simulink model "PID"  (R2019a)
settings: configuration reference "Configuration" (kept outside this file)
undefined symbols (not defined in the file): DiscIntNeverNeededParam, Model_Param
settings Model: Creator=zouji  LastModifiedBy=Bingo
settings ConfigSetRef: SourceName=Configuration  SourceLocation=Base Workspace

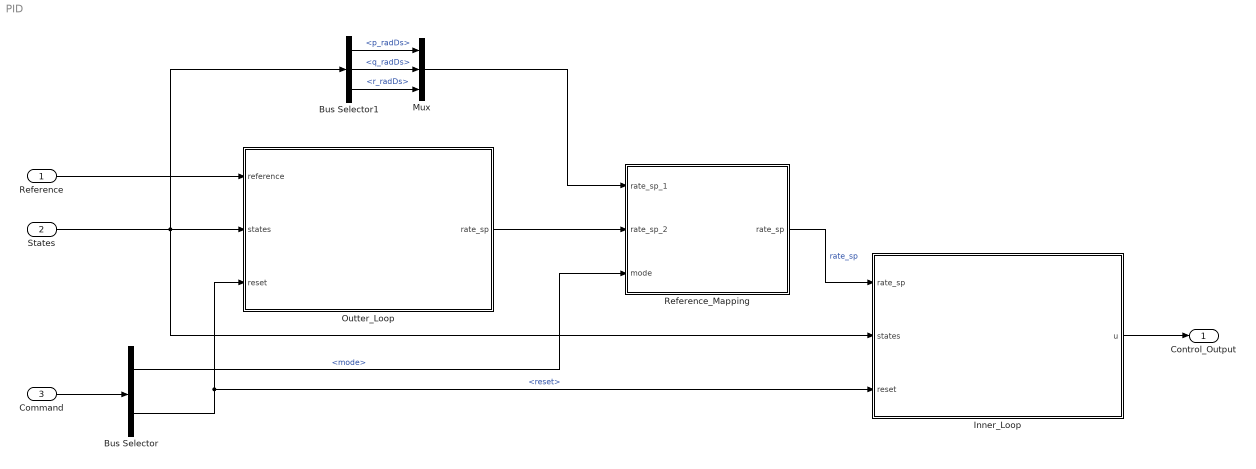
== system PID ==
  Reference : Inport  OutDataTypeStr=Bus: Reference
  States : Inport  Port=2  OutDataTypeStr=Bus: States
  Command : Inport  Port=3  OutDataTypeStr=Bus: Command
  Bus Selector : BusSelector  OutputSignals=mode,reset
  Bus Selector1 : BusSelector  OutputSignals=p_radDs,q_radDs,r_radDs
  Inner_Loop : Subsystem
  Mux : Mux  Inputs=3
  Outter_Loop : Subsystem
  Reference_Mapping : Subsystem
  Control_Output : Outport  OutDataTypeStr=Bus: Control_Output
  wires:
  Command/1 -> Bus Selector/1
  Reference/1 -> Outter_Loop/1(reference)
  States/1 -> Bus Selector1/1, Outter_Loop/2(states), Inner_Loop/2(states)
  Inner_Loop/1(u) -> Control_Output/1
  Bus Selector/2 -> Inner_Loop/3(reset), Outter_Loop/3(reset)  "<reset>"
  Reference_Mapping/1(rate_sp) -> Inner_Loop/1(rate_sp)  "rate_sp"
  Outter_Loop/1(rate_sp) -> Reference_Mapping/2(rate_sp_2)
  Bus Selector1/1 -> Mux/1  "<p_radDs>"
  Bus Selector1/2 -> Mux/2  "<q_radDs>"
  Bus Selector1/3 -> Mux/3  "<r_radDs>"
  Mux/1 -> Reference_Mapping/1(rate_sp_1)
  Bus Selector/1 -> Reference_Mapping/3(mode)  "<mode>"

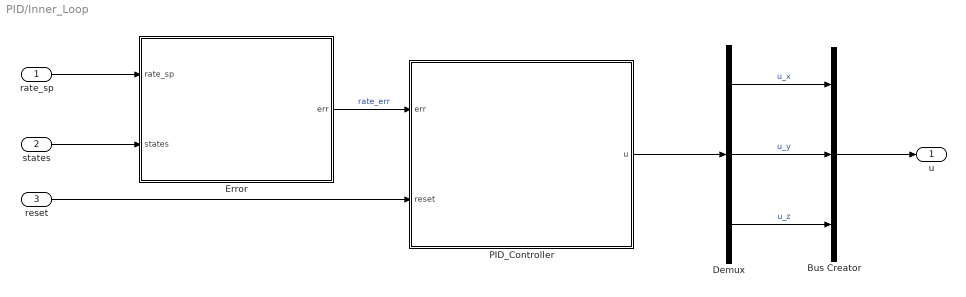
== system PID/Inner_Loop ==
  rate_sp : Inport
  states : Inport  Port=2
  reset : Inport  Port=3
  Bus Creator : BusCreator  Inputs=3
  Demux : Demux  Outputs=3
  Error : Subsystem
  PID_Controller : Subsystem
  u : Outport  OutDataTypeStr=Bus: Control_Output
  wires:
  states/1 -> Error/2(states)
  Error/1(err) -> PID_Controller/1(err)  "rate_err"
  rate_sp/1 -> Error/1(rate_sp)
  reset/1 -> PID_Controller/2(reset)
  PID_Controller/1(u) -> Demux/1
  Demux/1 -> Bus Creator/1  "u_x"
  Demux/2 -> Bus Creator/2  "u_y"
  Demux/3 -> Bus Creator/3  "u_z"
  Bus Creator/1 -> u/1

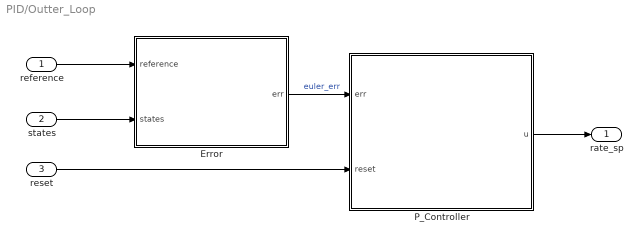
== system PID/Outter_Loop ==
  reference : Inport
  states : Inport  Port=2
  reset : Inport  Port=3
  Error : Subsystem
  P_Controller : Subsystem
  rate_sp : Outport
  wires:
  states/1 -> Error/2(states)
  Error/1(err) -> P_Controller/1(err)  "euler_err"
  P_Controller/1(u) -> rate_sp/1
  reset/1 -> P_Controller/2(reset)
  reference/1 -> Error/1(reference)

== system PID/Reference_Mapping ==
  note: mode=0, 外环输出作为目标角速度
      | mode=1, 输入指令作为目标角速度
  rate_sp_1 : Inport
  rate_sp_2 : Inport  Port=2
  mode : Inport  Port=3
  Switch : Switch  Criteria=u2 > Threshold
  rate_sp : Outport
  wires:
  mode/1 -> Switch/2
  rate_sp_1/1 -> Switch/1
  rate_sp_2/1 -> Switch/3
  Switch/1 -> rate_sp/1

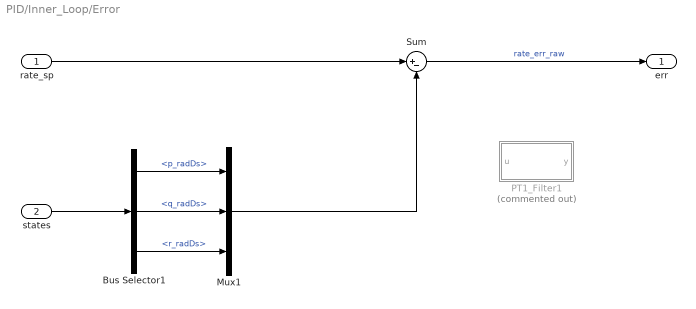
== system PID/Inner_Loop/Error ==
  rate_sp : Inport
  states : Inport  Port=2
  Bus Selector1 : BusSelector  OutputSignals=p_radDs,q_radDs,r_radDs
  Mux1 : Mux  Inputs=3
  PT1_Filter1 : Subsystem  Commented=on  mask{T_filter=0.05}
      mask prompts: T_filter "Time constant [s]"
      mask Display: fprintf('T = %.3f', T_filter)
  Sum : Sum  Inputs=|+-
  err : Outport
  wires:
  Bus Selector1/2 -> Mux1/2  "<q_radDs>"
  Bus Selector1/3 -> Mux1/3  "<r_radDs>"
  Bus Selector1/1 -> Mux1/1  "<p_radDs>"
  states/1 -> Bus Selector1/1
  Mux1/1 -> Sum/2
  Sum/1 -> err/1  "rate_err_raw"
  rate_sp/1 -> Sum/1

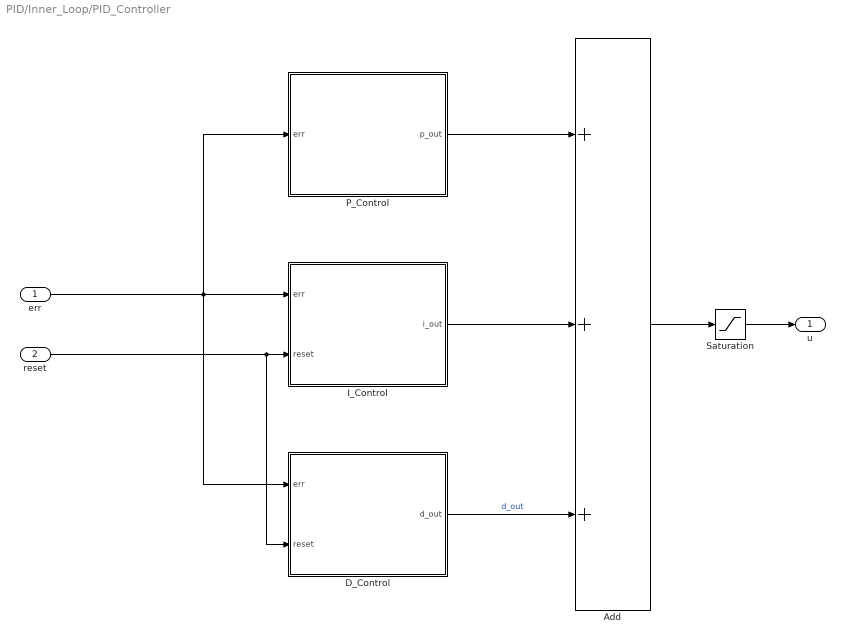
== system PID/Inner_Loop/PID_Controller ==
  err : Inport
  reset : Inport  Port=2
  Add : Sum  Inputs=+++
  D_Control : Subsystem  mask{p_kd=Model_Param.Kd_p, q_kd=Model_Param.Kd_q, r_kd=Model_Param.Kd_r, max_d=Model_Param.Kd_Max, min_d=Model_Param.Kd_Min}
  I_Control : Subsystem  mask{p_ki=Model_Param.Ki_p, q_ki=Model_Param.Ki_q, r_ki=Model_Param.Ki_r, max_i=Model_Param.Ki_Max, min_i=Model_Param.Ki_Min}
  P_Control : Subsystem  mask{p_kp=Model_Param.Kp_p, q_kp=Model_Param.Kp_q, r_kp=Model_Param.Kp_r}
  Saturation : Saturate  UpperLimit=1  LowerLimit=-1
  u : Outport
  wires:
  err/1 -> P_Control/1(err), I_Control/1(err), D_Control/1(err)
  P_Control/1(p_out) -> Add/1
  I_Control/1(i_out) -> Add/2
  D_Control/1(d_out) -> Add/3  "d_out"
  Saturation/1 -> u/1
  reset/1 -> I_Control/2(reset), D_Control/2(reset)
  Add/1 -> Saturation/1

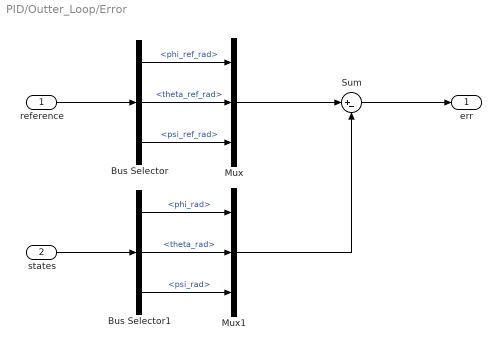
== system PID/Outter_Loop/Error ==
  reference : Inport
  states : Inport  Port=2
  Bus Selector : BusSelector  OutputSignals=phi_ref_rad,theta_ref_rad,psi_ref_rad
  Bus Selector1 : BusSelector  OutputSignals=phi_rad,theta_rad,psi_rad
  Mux : Mux  Inputs=3
  Mux1 : Mux  Inputs=3
  Sum : Sum  Inputs=|+-
  err : Outport
  wires:
  Bus Selector/3 -> Mux/3  "<psi_ref_rad>"
  Bus Selector1/2 -> Mux1/2  "<theta_rad>"
  Bus Selector/2 -> Mux/2  "<theta_ref_rad>"
  Bus Selector1/3 -> Mux1/3  "<psi_rad>"
  Bus Selector1/1 -> Mux1/1  "<phi_rad>"
  states/1 -> Bus Selector1/1
  Bus Selector/1 -> Mux/1  "<phi_ref_rad>"
  Mux1/1 -> Sum/2
  reference/1 -> Bus Selector/1
  Sum/1 -> err/1
  Mux/1 -> Sum/1

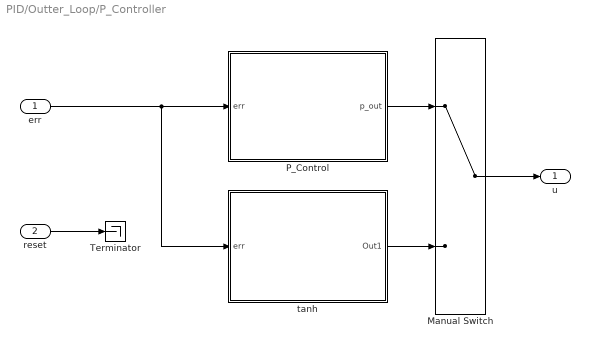
== system PID/Outter_Loop/P_Controller ==
  err : Inport
  reset : Inport  Port=2
  Manual Switch : ManualSwitch
  P_Control : Subsystem  mask{Kp_phi=Model_Param.Kp_phi, Kp_theta=Model_Param.Kp_theta, Kp_psi=Model_Param.Kp_psi}
  Terminator : Terminator
  tanh : Subsystem
  u : Outport
  wires:
  err/1 -> P_Control/1(err), tanh/1(err)
  reset/1 -> Terminator/1
  P_Control/1(p_out) -> Manual Switch/1
  tanh/1(Out1) -> Manual Switch/2
  Manual Switch/1 -> u/1

== system PID/Inner_Loop/Error/PT1_Filter1 ==
  u : Inport
  Discrete-Time Integrator1 : DiscreteIntegrator  InitialConditionSource=external  SampleTime=-1  OutDataTypeStr=single  ICPrevOutput=DiscIntNeverNeededParam  ICPrevScaledInput=DiscIntNeverNeededParam
  Sum5 : Sum  Inputs=|+-
  k_pt : Gain  Gain=1/T_filter
  y : Outport
  wires:
  k_pt/1 -> Discrete-Time Integrator1/1
  Discrete-Time Integrator1/1 -> Sum5/2, y/1
  Sum5/1 -> k_pt/1
  u/1 -> Sum5/1, Discrete-Time Integrator1/2

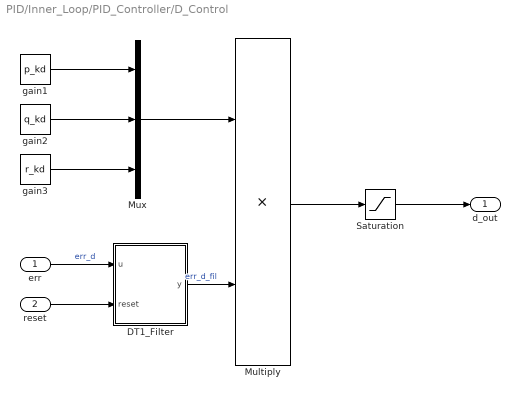
== system PID/Inner_Loop/PID_Controller/D_Control ==
  err : Inport
  reset : Inport  Port=2
  DT1_Filter : Subsystem  mask{T_filter=0.02}
      mask prompts: T_filter "Time constant [s]"
      mask Display: fprintf('T = %.3f', T_filter)
  Multiply : Product  OutDataTypeStr=Inherit: Same as first input
  Mux : Mux  Inputs=3
  Saturation : Saturate  UpperLimit=max_d  LowerLimit=min_d
  gain1 : Constant  Value=p_kd  OutDataTypeStr=single
  gain2 : Constant  Value=q_kd  OutDataTypeStr=single
  gain3 : Constant  Value=r_kd  OutDataTypeStr=single
  d_out : Outport
  wires:
  err/1 -> DT1_Filter/1(u)  "err_d"
  gain2/1 -> Mux/2
  Mux/1 -> Multiply/1
  gain1/1 -> Mux/1
  Multiply/1 -> Saturation/1
  gain3/1 -> Mux/3
  DT1_Filter/1(y) -> Multiply/2  "err_d_fil"
  Saturation/1 -> d_out/1
  reset/1 -> DT1_Filter/2(reset)

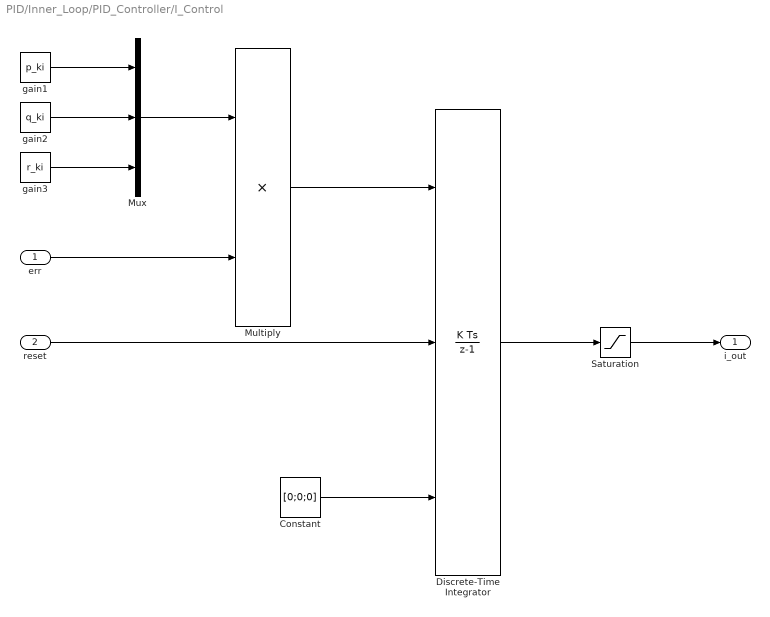
== system PID/Inner_Loop/PID_Controller/I_Control ==
  err : Inport
  reset : Inport  Port=2
  Constant : Constant  Value=[0;0;0]  OutDataTypeStr=single
  Discrete-Time Integrator : DiscreteIntegrator  ExternalReset=level  InitialConditionSource=external  SampleTime=-1  ICPrevOutput=DiscIntNeverNeededParam  ICPrevScaledInput=DiscIntNeverNeededParam
  Multiply : Product  OutDataTypeStr=Inherit: Same as first input
  Mux : Mux  Inputs=3
  Saturation : Saturate  UpperLimit=max_i  LowerLimit=min_i
  gain1 : Constant  Value=p_ki  OutDataTypeStr=single
  gain2 : Constant  Value=q_ki  OutDataTypeStr=single
  gain3 : Constant  Value=r_ki  OutDataTypeStr=single
  i_out : Outport
  wires:
  err/1 -> Multiply/2
  gain2/1 -> Mux/2
  Mux/1 -> Multiply/1
  gain1/1 -> Mux/1
  gain3/1 -> Mux/3
  Multiply/1 -> Discrete-Time Integrator/1
  reset/1 -> Discrete-Time Integrator/2
  Constant/1 -> Discrete-Time Integrator/3
  Discrete-Time Integrator/1 -> Saturation/1
  Saturation/1 -> i_out/1

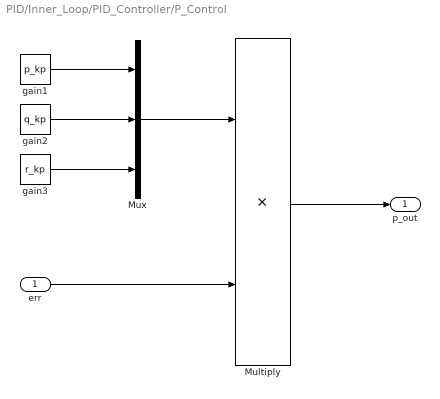
== system PID/Inner_Loop/PID_Controller/P_Control ==
  err : Inport
  Multiply : Product  OutDataTypeStr=Inherit: Same as first input
  Mux : Mux  Inputs=3
  gain1 : Constant  Value=p_kp  OutDataTypeStr=single
  gain2 : Constant  Value=q_kp  OutDataTypeStr=single
  gain3 : Constant  Value=r_kp  OutDataTypeStr=single
  p_out : Outport
  wires:
  err/1 -> Multiply/2
  gain2/1 -> Mux/2
  Mux/1 -> Multiply/1
  gain1/1 -> Mux/1
  Multiply/1 -> p_out/1
  gain3/1 -> Mux/3

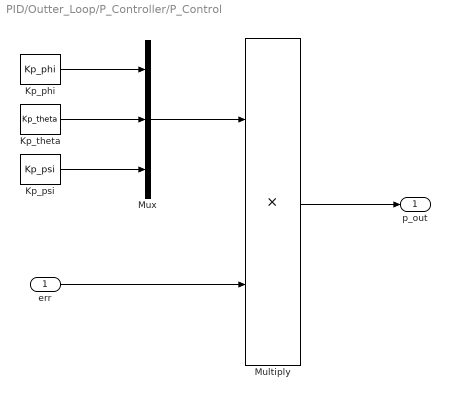
== system PID/Outter_Loop/P_Controller/P_Control ==
  err : Inport
  "Kp_phi " : Constant  Value=Kp_phi  OutDataTypeStr=single
  Kp_psi : Constant  Value=Kp_psi  OutDataTypeStr=single
  Kp_theta : Constant  Value=Kp_theta  OutDataTypeStr=single
  Multiply : Product  OutDataTypeStr=Inherit: Same as first input
  Mux : Mux  Inputs=3
  p_out : Outport
  wires:
  err/1 -> Multiply/2
  Kp_theta/1 -> Mux/2
  Mux/1 -> Multiply/1
  "Kp_phi "/1 -> Mux/1
  Multiply/1 -> p_out/1
  Kp_psi/1 -> Mux/3

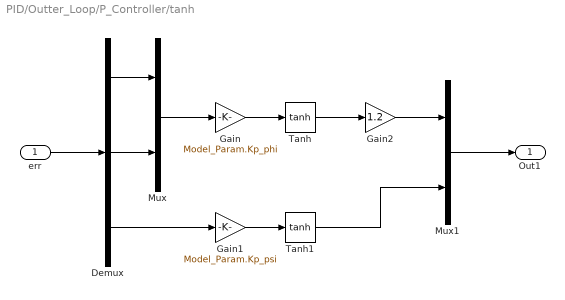
== system PID/Outter_Loop/P_Controller/tanh ==
  err : Inport
  Demux : Demux  Outputs=3
  Gain : Gain  Gain=Model_Param.Kp_phi
  Gain1 : Gain  Gain=Model_Param.Kp_psi
  Gain2 : Gain  Gain=1.2
  Mux : Mux  Inputs=2
  Mux1 : Mux  Inputs=2
  Tanh : Trigonometry  Operator=tanh
  Tanh1 : Trigonometry  Operator=tanh
  Out1 : Outport
  wires:
  Gain/1 -> Tanh/1
  err/1 -> Demux/1
  Demux/1 -> Mux/1
  Demux/2 -> Mux/2
  Mux/1 -> Gain/1
  Gain1/1 -> Tanh1/1
  Demux/3 -> Gain1/1
  Tanh/1 -> Gain2/1
  Gain2/1 -> Mux1/1
  Tanh1/1 -> Mux1/2
  Mux1/1 -> Out1/1

== system PID/Inner_Loop/PID_Controller/D_Control/DT1_Filter ==
  u : Inport
  reset : Inport  Port=2
  Discrete-Time Integrator1 : DiscreteIntegrator  ExternalReset=level  SampleTime=-1  ICPrevOutput=DiscIntNeverNeededParam  ICPrevScaledInput=DiscIntNeverNeededParam
  Sum5 : Sum  Inputs=|+-
  k_pt : Gain  Gain=1/T_filter  OutDataTypeStr=Inherit: Same as input
  y : Outport
  wires:
  u/1 -> Sum5/1
  Sum5/1 -> k_pt/1
  Discrete-Time Integrator1/1 -> Sum5/2
  k_pt/1 -> Discrete-Time Integrator1/1, y/1
  reset/1 -> Discrete-Time Integrator1/2
